simulink model "LongLatDriveline"  (R2024b)
settings: Solver=FixedStepAuto  StartTime=0  StopTime=120  FixedStep=0.002  RelTol=1e-3
InitFcn:
  | load('waypoints.mat');
  | VehicleObj = Simulink.data.dictionary.open('./ModelData/VehicleData.sldd');
  | %dDataSectObj = getSection(myDictionaryObj,'Design Data');
StopFcn:
  | Plot_LateralModelErrorControl;
  | 
  | mdlWks = get_param(gcs, 'ModelWorkspace');
  | par_ToDrvDesigner = evalin(mdlWks, 'ToDrvDesigner');
  | 
  | if par_ToDrvDesigner.Value
  |     ExportdrivingScenario;
  | end
model workspace (MAT data in the model file):
  ToDrvDesigner : Simulink.Parameter (value not decoded)
values from neighbouring files (symbols this model uses):
  A_F = 2.341157    [VehicleData.sldd]
  C_af = 80000.0    [VehicleData.sldd]
  C_ar = 80000.0    [VehicleData.sldd]
  C_d = 0.24    [VehicleData.sldd]
  f = 0.01    [VehicleData.sldd]
  g = 9.81    [VehicleData.sldd]
  h_aero = 0.65    [VehicleData.sldd]
  h_gc = 0.65    [VehicleData.sldd]
  Iz = 2873.0    [VehicleData.sldd]
  lf = 1.1    [VehicleData.sldd]
  lr = 1.58    [VehicleData.sldd]
  m = 2238.932    [VehicleData.sldd]
  Nf = 2.0    [VehicleData.sldd]
  Nr = 2.0    [VehicleData.sldd]
  r_stat = 0.342    [VehicleData.sldd]
  r_w = 0.352    [VehicleData.sldd]
  rho = 1.225    [VehicleData.sldd]
  theta = 0.0    [VehicleData.sldd]
  transGear = 0.1027    [VehicleData.sldd]
  V_wind = 0.0    [VehicleData.sldd]
symbols that are objects in the model workspace (value not decoded): ToDrvDesigner
undefined symbols (not defined in the file or in its folder): InitialPsi, InitialX, InitialY, phi
libraries: slpidlib x14, spsMosfetLib x6, simulink x4, spsVoltageMeasurementLib x3, SignalEditorBlockLib x2, spsDCVoltageSourceLib x1, spspowerguiLib x1
(part 2 of 5)

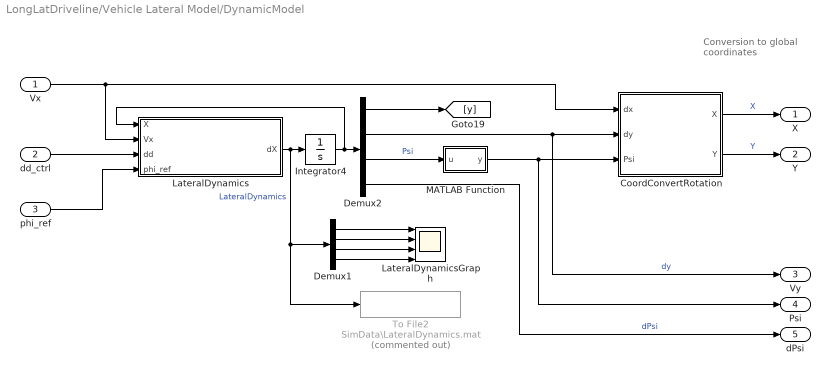
== system LongLatDriveline/Vehicle Lateral Model/DynamicModel ==
  note: Conversion to global
      | coordinates
  Vx : Inport
  dd_ctrl : Inport  Port=2
  phi_ref : Inport  Port=3
  CoordConvertRotation : Subsystem
      mask Display: image('rotatingFrame.png');
  Demux1 : Demux
  Demux2 : Demux
  Integrator4 : Integrator  InitialCondition=[0;0;InitialPsi;0.0423]
  LateralDynamics : Subsystem  Variant=on  VariantControlMode=label  LabelModeActiveChoice=Not Simplified Model
  LateralDynamicsGraph : Scope  NumInputPorts=4
  MATLAB Function : MATLAB Function  TreatAsAtomicUnit=on
  To File2 : ToFile  Commented=on  Filename=SimData\LateralDynamics.mat  SaveFormat=Timeseries
  X : Outport
  Y : Outport  Port=2
  Vy : Outport  Port=3
  Psi : Outport  Port=4
  dPsi : Outport  Port=5
  wires:
  Integrator4/1 -> LateralDynamics/1(X), Demux2/1
  phi_ref/1 -> LateralDynamics/4(phi_ref)
  Demux2/2 -> Vy/1, CoordConvertRotation/2(dy)  "dy"
  Demux1/1 -> LateralDynamicsGraph/1
  LateralDynamics/1(dX) -> To File2/1, Demux1/1, Integrator4/1  "LateralDynamics"
  Demux2/3 -> MATLAB Function/1(u)  "Psi"
  Vx/1 -> CoordConvertRotation/1(dx), LateralDynamics/2(Vx)
  Demux1/2 -> LateralDynamicsGraph/2
  CoordConvertRotation/1(X) -> X/1  "X"
  Demux1/4 -> LateralDynamicsGraph/4
  Demux2/1 -> [y]
  Demux1/3 -> LateralDynamicsGraph/3
  CoordConvertRotation/2(Y) -> Y/1  "Y"
  dd_ctrl/1 -> LateralDynamics/3(dd)
  MATLAB Function/1(y) -> CoordConvertRotation/3(Psi), Psi/1
  Demux2/4 -> dPsi/1  "dPsi"

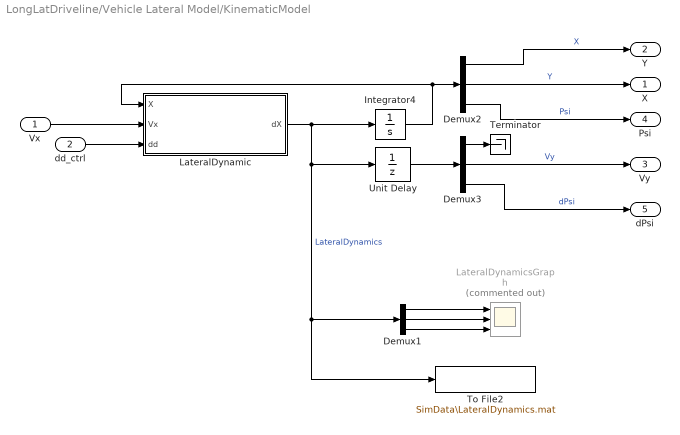
== system LongLatDriveline/Vehicle Lateral Model/KinematicModel ==
  Vx : Inport
  dd_ctrl : Inport  Port=2
  Demux1 : Demux  Outputs=3
  Demux2 : Demux  Outputs=3
  Demux3 : Demux  Outputs=3
  Integrator4 : Integrator  InitialCondition=[InitialY;InitialX;InitialPsi]
  LateralDynamic : MATLAB Function  TreatAsAtomicUnit=on  VariantControl=Simplified Model
  LateralDynamicsGraph : Scope  Commented=on  NumInputPorts=3
  Terminator : Terminator
  To File2 : ToFile  Filename=SimData\LateralDynamics.mat  SaveFormat=Timeseries
  Unit Delay : UnitDelay  InitialCondition=[0;0;0]  SampleTime=-1  HasFrameUpgradeWarning=on
  X : Outport
  Y : Outport  Port=2
  Vy : Outport  Port=3
  Psi : Outport  Port=4
  dPsi : Outport  Port=5
  wires:
  Integrator4/1 -> LateralDynamic/1(X), Demux2/1
  Vx/1 -> LateralDynamic/2(Vx)
  Demux1/1 -> LateralDynamicsGraph/1
  dd_ctrl/1 -> LateralDynamic/3(dd)
  LateralDynamic/1(dX) -> Integrator4/1, Unit Delay/1, Demux1/1, To File2/1  "LateralDynamics"
  Demux1/3 -> LateralDynamicsGraph/3
  Demux1/2 -> LateralDynamicsGraph/2
  Demux2/1 -> Y/1  "X"
  Demux2/2 -> X/1  "Y"
  Demux2/3 -> Psi/1  "Psi"
  Demux3/3 -> dPsi/1  "dPsi"
  Demux3/2 -> Vy/1  "Vy"
  Demux3/1 -> Terminator/1
  Unit Delay/1 -> Demux3/1

== system LongLatDriveline/LateralController/SMC_Alcala/LevantDiff ==
  X : Inport
  Constant : Constant  Value=lambda1
  Constant1 : Constant  Value=alpha1
  Demux : Demux  Outputs=2
  Integrator : Integrator  InitialCondition=[0 0]
  Levant : MATLAB Function  TreatAsAtomicUnit=on
  Terminator : Terminator
  dX : Outport  VectorParamsAs1DForOutWhenUnconnected=off
  wires:
  X/1 -> Levant/2(u_ref)
  Levant/1(dX) -> Integrator/1, Demux/1
  Integrator/1 -> Levant/1(X)
  Constant/1 -> Levant/3(lambda)
  Constant1/1 -> Levant/4(alpha)
  Demux/1 -> dX/1
  Demux/2 -> Terminator/1

== system LongLatDriveline/LateralController/SMC_Alcala/LevantDiff1 ==
  X : Inport
  Constant : Constant  Value=lambda1
  Constant1 : Constant  Value=alpha1
  Demux : Demux  Outputs=2
  Integrator : Integrator  InitialCondition=[0 0]
  Levant : MATLAB Function  TreatAsAtomicUnit=on
  Terminator : Terminator
  dX : Outport  VectorParamsAs1DForOutWhenUnconnected=off
  wires:
  X/1 -> Levant/2(u_ref)
  Levant/1(dX) -> Integrator/1, Demux/1
  Integrator/1 -> Levant/1(X)
  Constant/1 -> Levant/3(lambda)
  Constant1/1 -> Levant/4(alpha)
  Demux/1 -> dX/1
  Demux/2 -> Terminator/1

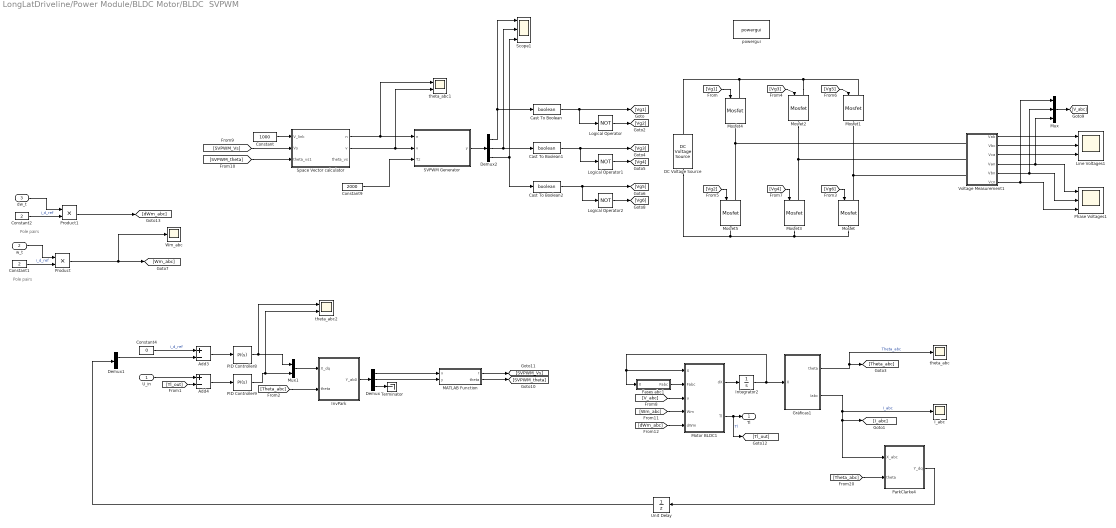
== system LongLatDriveline/Power Module/BLDC Motor/BLDC  SVPWM ==
  note: Pole pairs
  note: Pole pairs
  U_in : Inport
  w_t : Inport  Port=2
  dw_t : Inport  Port=3
  Add3 : Sum  Inputs=+-
  Add4 : Sum  Inputs=+-
  Cast To Boolean : DataTypeConversion  OutDataTypeStr=boolean  SaturateOnIntegerOverflow=off  RndMeth=Floor
  Cast To Boolean1 : DataTypeConversion  OutDataTypeStr=boolean  SaturateOnIntegerOverflow=off  RndMeth=Floor
  Cast To Boolean2 : DataTypeConversion  OutDataTypeStr=boolean  SaturateOnIntegerOverflow=off  RndMeth=Floor
  Constant : Constant  Value=1000
  Constant1 : Constant  Value=2
  Constant2 : Constant  Value=2
  Constant4 : Constant  Value=0
  Constant9 : Constant  Value=2000
  DC Voltage Source : spsDCVoltageSourceLib/DC Voltage Source  Amplitude=1000  Measurements=None
  Demux : Demux  Outputs=3
  Demux1 : Demux  Outputs=2
  Demux2 : Demux  Outputs=3
  Fases abc1 : MATLAB Function  TreatAsAtomicUnit=on
  Gráficas1 : MATLAB Function  TreatAsAtomicUnit=on
  I_abc : Scope
  Integrator2 : Integrator  InitialCondition=[0 0 0 0]
  InvPark : MATLAB Function  TreatAsAtomicUnit=on
  Line Voltages1 : Scope  NumInputPorts=3
  Logical Operator : Logic  Operator=NOT  IconShape=distinctive  AllPortsSameDT=off  OutDataTypeStr=boolean
  Logical Operator1 : Logic  Operator=NOT  IconShape=distinctive  AllPortsSameDT=off  OutDataTypeStr=boolean
  Logical Operator2 : Logic  Operator=NOT  IconShape=distinctive  AllPortsSameDT=off  OutDataTypeStr=boolean
  MATLAB Function : MATLAB Function  TreatAsAtomicUnit=on
  Mosfet{,1..5} (6 alike) : spsMosfetLib/Mosfet  Ron=0.1  Lon=0  Rd=0.01  Vfd=0  IC=0  Rs=1e5  Cs=inf  Measurements=off
  Motor BLDC1 : MATLAB Function  TreatAsAtomicUnit=on
  Mux : Mux  Inputs=3
  Mux1 : Mux  Inputs=2
  PID Controller8 : slpidlib/PID Controller  Controller=PI  Form=Parallel  TimeDomain=Continuous-time  UseExternalTs=off  SampleTime=-1  IntegratorMethod=Forward Euler  FilterMethod=Forward Euler  ControllerParametersSource=internal  P=0.203768519261034  I=30.7991199051557  UseKiTs=off  D=-6.74177637974606e-05  UseExternalDerivativeSource=off  N=1209.06435302465  UseFilter=on  TunerSelectOption=Transfer Function Based (PID Tuner App)  InitialConditionSource=internal  InitialConditionForIntegrator=0  InitialConditionForFilter=0  DifferentiatorICPrevScaledInput=0  ExternalReset=none  TrackingMode=off  Kt=1  LimitOutput=off  SatLimitsSource=internal  UpperSaturationLimit=inf  LowerSaturationLimit=-inf  LinearizeAsGain=on  AntiWindupMode=none  Kb=1  LimitIntegrator=off  UpperIntegratorSaturationLimit=inf  LowerIntegratorSaturationLimit=-inf  POutMin=[]  POutMax=[]  IOutMin=[]  IOutMax=[]  DOutMin=[]  DOutMax=[]  NOutMin=[]  NOutMax=[]  SumOutMin=[]  SumOutMax=[]  SaturationOutMin=[]  SaturationOutMax=[]  PParamMin=[]  PParamMax=[]  IParamMin=[]  IParamMax=[]  DParamMin=[]  DParamMax=[]  NParamMin=[]  NParamMax=[]  KbParamMin=[]  KbParamMax=[]  KtParamMin=[]  KtParamMax=[]  KbOutMin=[]  KbOutMax=[]  KtOutMin=[]  KtOutMax=[]  IntegratorOutMin=[]  IntegratorOutMax=[]  FilterOutMin=[]  FilterOutMax=[]  SumI1OutMin=[]  SumI1OutMax=[]  SumI2OutMin=[]  SumI2OutMax=[]  SumI3OutMin=[]  SumI3OutMax=[]  SumI4OutMin=[]  SumI4OutMax=[]  SumDOutMin=[]  SumDOutMax=[]  DifferentiatorOutMin=[]  DifferentiatorOutMax=[]  FilterDiffOutCoefMin=[]  FilterDiffOutCoefMax=[]  ReciprocalOutMin=[]  ReciprocalOutMax=[]  SumDenOutMin=[]  SumDenOutMax=[]  SumNumOutMin=[]  SumNumOutMax=[]  DivideOutMin=[]  DivideOutMax=[]  UdiffTsProdOutMin=[]  UdiffTsProdOutMax=[]  NTsProdOutMin=[]  NTsProdOutMax=[]  UintegralTsProdOutMin=[]  UintegralTsProdOutMax=[]  UngainTsProdOutMin=[]  UngainTsProdOutMax=[]  ClampingZeroOutDataTypeStr=Inherit: Inherit via back propagation  ClampingZeroOutMin=[]  ClampingZeroOutMax=[]  FilterDenConstantOutDataTypeStr=Inherit: Inherit via back propagation  FilterDenConstantOutMin=[]  FilterDenConstantOutMax=[]  PCopyOutDataTypeStr=Inherit: Inherit via back propagation  PCopyOutMin=[]  PCopyOutMax=[]  NCopyOutDataTypeStr=Inherit: Inherit via back propagation  NCopyOutMin=[]  NCopyOutMax=[]  IntegratorContinuousStateAttributes=''  IntegratorStateMustResolveToSignalObject=off  IntegratorRTWStateStorageClass=Auto  FilterContinuousStateAttributes=''  FilterStateMustResolveToSignalObject=off  FilterRTWStateStorageClass=Auto  ParallelPVariant=InternalParameters  IdealPVariant=Disabled  IVariant=InternalParameters  DVariant=Disabled  IntegratorVariant=Continuous  SatVariant=Disabled  AWVariant=Passthrough  PCopyVariant=Disabled  TRVariant=Disabled  FdbkBlocksVariant=Forward  IdealPFdbkVariant=Disabled  SatFdbkVariant=Disabled  DerivativeFilterVariant=Disabled  NVariant=Disabled  NCopyVariant=Disabled_SignalSpec  FilterICVariant=Disabled  IntegratorICVariant=InternalICs  ExternalResetVariant=Disabled  TRSumVariant=Passthrough  SumFdbkVariant=Disabled  SumVariant=Sum_PI  TsampFilterVariant=InternalTs  TsampNgainVariant=Passthrough  TsampIntegralVariant=Disabled_SignalSpec  ExternalSaturationOutDataTypeStr=Inherit: Same as second input  DerivativeSourceVariant=Disabled  PreIntVariant=InternalPreInt
  PID Controller9 : slpidlib/PID Controller  Controller=PI  Form=Parallel  TimeDomain=Continuous-time  UseExternalTs=off  SampleTime=-1  IntegratorMethod=Forward Euler  FilterMethod=Forward Euler  ControllerParametersSource=internal  P=0.203768519261034  I=30.7991199051557  UseKiTs=off  D=-6.74177637974606e-05  UseExternalDerivativeSource=off  N=1209.06435302465  UseFilter=on  TunerSelectOption=Transfer Function Based (PID Tuner App)  InitialConditionSource=internal  InitialConditionForIntegrator=0  InitialConditionForFilter=0  DifferentiatorICPrevScaledInput=0  ExternalReset=none  TrackingMode=off  Kt=1  LimitOutput=off  SatLimitsSource=internal  UpperSaturationLimit=inf  LowerSaturationLimit=-inf  LinearizeAsGain=on  AntiWindupMode=none  Kb=1  LimitIntegrator=off  UpperIntegratorSaturationLimit=inf  LowerIntegratorSaturationLimit=-inf  POutMin=[]  POutMax=[]  IOutMin=[]  IOutMax=[]  DOutMin=[]  DOutMax=[]  NOutMin=[]  NOutMax=[]  SumOutMin=[]  SumOutMax=[]  SaturationOutMin=[]  SaturationOutMax=[]  PParamMin=[]  PParamMax=[]  IParamMin=[]  IParamMax=[]  DParamMin=[]  DParamMax=[]  NParamMin=[]  NParamMax=[]  KbParamMin=[]  KbParamMax=[]  KtParamMin=[]  KtParamMax=[]  KbOutMin=[]  KbOutMax=[]  KtOutMin=[]  KtOutMax=[]  IntegratorOutMin=[]  IntegratorOutMax=[]  FilterOutMin=[]  FilterOutMax=[]  SumI1OutMin=[]  SumI1OutMax=[]  SumI2OutMin=[]  SumI2OutMax=[]  SumI3OutMin=[]  SumI3OutMax=[]  SumI4OutMin=[]  SumI4OutMax=[]  SumDOutMin=[]  SumDOutMax=[]  DifferentiatorOutMin=[]  DifferentiatorOutMax=[]  FilterDiffOutCoefMin=[]  FilterDiffOutCoefMax=[]  ReciprocalOutMin=[]  ReciprocalOutMax=[]  SumDenOutMin=[]  SumDenOutMax=[]  SumNumOutMin=[]  SumNumOutMax=[]  DivideOutMin=[]  DivideOutMax=[]  UdiffTsProdOutMin=[]  UdiffTsProdOutMax=[]  NTsProdOutMin=[]  NTsProdOutMax=[]  UintegralTsProdOutMin=[]  UintegralTsProdOutMax=[]  UngainTsProdOutMin=[]  UngainTsProdOutMax=[]  ClampingZeroOutDataTypeStr=Inherit: Inherit via back propagation  ClampingZeroOutMin=[]  ClampingZeroOutMax=[]  FilterDenConstantOutDataTypeStr=Inherit: Inherit via back propagation  FilterDenConstantOutMin=[]  FilterDenConstantOutMax=[]  PCopyOutDataTypeStr=Inherit: Inherit via back propagation  PCopyOutMin=[]  PCopyOutMax=[]  NCopyOutDataTypeStr=Inherit: Inherit via back propagation  NCopyOutMin=[]  NCopyOutMax=[]  IntegratorContinuousStateAttributes=''  IntegratorStateMustResolveToSignalObject=off  IntegratorRTWStateStorageClass=Auto  FilterContinuousStateAttributes=''  FilterStateMustResolveToSignalObject=off  FilterRTWStateStorageClass=Auto  ParallelPVariant=InternalParameters  IdealPVariant=Disabled  IVariant=InternalParameters  DVariant=Disabled  IntegratorVariant=Continuous  SatVariant=Disabled  AWVariant=Passthrough  PCopyVariant=Disabled  TRVariant=Disabled  FdbkBlocksVariant=Forward  IdealPFdbkVariant=Disabled  SatFdbkVariant=Disabled  DerivativeFilterVariant=Disabled  NVariant=Disabled  NCopyVariant=Disabled_SignalSpec  FilterICVariant=Disabled  IntegratorICVariant=InternalICs  ExternalResetVariant=Disabled  TRSumVariant=Passthrough  SumFdbkVariant=Disabled  SumVariant=Sum_PI  TsampFilterVariant=InternalTs  TsampNgainVariant=Passthrough  TsampIntegralVariant=Disabled_SignalSpec  ExternalSaturationOutDataTypeStr=Inherit: Same as second input  DerivativeSourceVariant=Disabled  PreIntVariant=InternalPreInt
  ParkClarke4 : MATLAB Function  TreatAsAtomicUnit=on
  Phase Voltages1 : Scope  NumInputPorts=3
  Product : Product
  Product1 : Product
  SVPWM Generator : Subsystem
  Scope1 : Scope  NumInputPorts=3
  Space Vector calculator : MATLAB Function  TreatAsAtomicUnit=on
  Terminator : Terminator
  Unit Delay : UnitDelay  SampleTime=-1  HasFrameUpgradeWarning=on
  Voltage Measurement1 : Subsystem
  Wm_abc : Scope
  powergui : spspowerguiLib/powergui  Priority=1  SimulationMode=Discrete  SampleTime=2e-6  frequency=60  Iterations=50  frequencyindice=0  Pbase=100e6  ErrMax=1e-4  UnitsV=kV  UnitsW=MW  buscounter=0  FunctionMessages=off  echomessages=off  EnableUseOfTLC=off  CurrentSourceSwitches=off  DisableSnubberDevices=off  DisableRonSwitches=off  DisableVfSwitches=off  DisplayEquations=off  AutomaticDiscreteSolvers=off  SolverType=Tustin/Backward Euler (TBE)  Interpol=off  ExternalGateDelay=off  methode=off  Ts=100  x0status=blocks  SPID=off  SwTol=0  HookPort=off  NonlinearTolerance=1e-4  nMaxIteration=100  ContinueOnMaxIteration=off  RestoreLinks=warning  ResistiveCurrentMeasurement=off  Frange=[0:2:500]  Ylog=off  Xlog=on  ShowGrid=off  save=off  variable=ZData  structure=ScopeData3  ZoomFFT=off  StartTime=0.04  cycles=1  DisplayStyle=1  fundamental=50  FreqAxis=off  MaxFrequency=2000  frequencyindicesteady=1  RmsSteady=1  display=off
  theta_abc : Scope
  theta_abc1 : Scope  NumInputPorts=2
  theta_abc2 : Scope  NumInputPorts=2
  Tl : Outport
  wires:
  MATLAB Function/2(theta) -> [SVPWM_theta]
  Voltage Measurement1/6(Vcn) -> Mux/1, Phase Voltages1/3
  Demux/1 -> MATLAB Function/1(x)
  Add4/1 -> PID Controller9/1
  Space Vector calculator/2(v) -> SVPWM Generator/2(v), theta_abc1/2
  Demux1/1 -> Add3/2
  [SVPWM_Vs] -> Space Vector calculator/2(Vs)
  Cast To Boolean/1 -> Logical Operator/1, [Vg1]
  SVPWM Generator/1(y) -> Demux2/1
  Logical Operator2/1 -> [Vg6]
  [SVPWM_theta] -> Space Vector calculator/3(theta_vs1)
  Cast To Boolean1/1 -> Logical Operator1/1, [Vg3]
  MATLAB Function/1(r) -> [SVPWM_Vs]
  Voltage Measurement1/2(Vbc) -> Line Voltages1/2
  Mux1/1 -> InvPark/1(X_dq)
  Logical Operator/1 -> [Vg2]
  Logical Operator1/1 -> [Vg4]
  [Theta_abc] -> InvPark/2(theta)
  Demux/3 -> Terminator/1
  Cast To Boolean2/1 -> Logical Operator2/1, [Vg5]
  Demux2/1 -> Cast To Boolean/1, Scope1/1
  [Vg2] -> Mosfet5/1
  Demux/2 -> MATLAB Function/2(y)
  [Vg1] -> Mosfet4/1
  Constant/1 -> Space Vector calculator/1(V_link)
  Mux/1 -> [V_abc]
  Gráficas1/2(Iabc) -> ParkClarke4/1(X_abc), [I_abc], I_abc/1  "I_abc"
  Voltage Measurement1/4(Van) -> Mux/3, Phase Voltages1/1
  Voltage Measurement1/5(Vbn) -> Mux/2, Phase Voltages1/2
  [Vg3] -> Mosfet2/1
  [Vg5] -> Mosfet1/1
  Space Vector calculator/1(n) -> SVPWM Generator/1(n), theta_abc1/1
  Constant9/1 -> SVPWM Generator/3(Tz)
  ParkClarke4/1(Y_dq) -> Unit Delay/1
  Demux2/3 -> Cast To Boolean2/1, Scope1/3
  [Vg6] -> Mosfet/1
  Voltage Measurement1/3(Vca) -> Line Voltages1/3
  Demux2/2 -> Cast To Boolean1/1, Scope1/2
  [Theta_abc] -> ParkClarke4/2(theta)
  Gráficas1/1(theta) -> theta_abc/1, [Theta_abc]  "Theta_abc"
  [Vg4] -> Mosfet3/1
  Voltage Measurement1/1(Vab) -> Line Voltages1/1
  Add3/1 -> PID Controller8/1
  Unit Delay/1 -> Demux1/1
  PID Controller9/1 -> Mux1/2, theta_abc2/2
  PID Controller8/1 -> Mux1/1, theta_abc2/1
  Integrator2/1 -> Gráficas1/1(X), Motor BLDC1/1(X), Fases abc1/1(X)
  Constant4/1 -> Add3/1  "i_d_ref"
  InvPark/1(Y_ab0) -> Demux/1
  Motor BLDC1/1(dX) -> Integrator2/1
  [V_abc] -> Motor BLDC1/3(u)
  Fases abc1/1(Fabc) -> Motor BLDC1/2(Fabc)
  Motor BLDC1/2(Tl) -> [Tl_out], Tl/1  "Tl"
  [Wm_abc] -> Motor BLDC1/4(Wm)
  U_in/1 -> Add4/1
  [Tl_out] -> Add4/2
  w_t/1 -> Product/1
  Constant1/1 -> Product/2  "i_d_ref"
  Product/1 -> Wm_abc/1, [Wm_abc]
  Constant2/1 -> Product1/2  "i_d_ref"
  dw_t/1 -> Product1/1
  Product1/1 -> [dWm_abc]
  [dWm_abc] -> Motor BLDC1/5(dWm)
  connections:
  DC Voltage Source/LConn1 -- Mosfet3/RConn1 -- Mosfet/RConn1 -- Mosfet5/RConn1
  Mosfet4/RConn1 -- Mosfet5/LConn1 -- Voltage Measurement1/LConn1
  Mosfet2/LConn1 -- Mosfet1/LConn1 -- DC Voltage Source/RConn1 -- Mosfet4/LConn1
  Mosfet1/RConn1 -- Voltage Measurement1/LConn3 -- Mosfet/LConn1
  Mosfet2/RConn1 -- Voltage Measurement1/LConn2 -- Mosfet3/LConn1

== system LongLatDriveline/Power Module/BLDC Motor/BLDC abcModel ==
  U_in : Inport
  w_t : Inport  Port=2
  dw_t : Inport  Port=3
  Fases abc : MATLAB Function  TreatAsAtomicUnit=on
  Graphs : MATLAB Function  TreatAsAtomicUnit=on
  Iabc : Scope
  Integrator2 : Integrator  InitialCondition=[0 0 0 0]
  Motor BLDC : MATLAB Function  TreatAsAtomicUnit=on
  theta : Scope
  Tl : Outport
  wires:
  Graphs/1(theta) -> theta/1
  Graphs/2(Iabc) -> Iabc/1
  Fases abc/1(Fabc) -> Motor BLDC/2(Fabc)
  Motor BLDC/1(dX) -> Integrator2/1
  Integrator2/1 -> Graphs/1(X), Motor BLDC/1(X), Fases abc/1(X)
  Motor BLDC/2(Tl) -> Tl/1  "Tl"
  dw_t/1 -> Motor BLDC/5(dWm)
  w_t/1 -> Motor BLDC/4(Wm)
  U_in/1 -> Motor BLDC/3(u)  "i_q_ref"

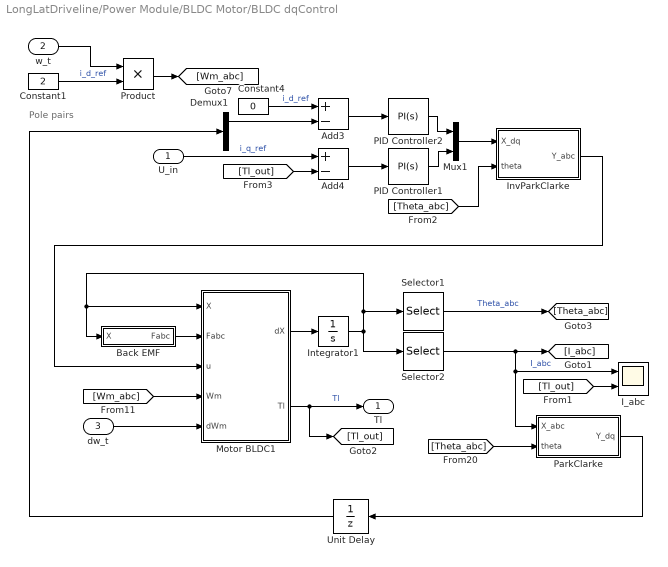
== system LongLatDriveline/Power Module/BLDC Motor/BLDC dqControl ==
  note: Pole pairs
  U_in : Inport
  w_t : Inport  Port=2
  dw_t : Inport  Port=3
  Add3 : Sum  Inputs=+-
  Add4 : Sum  Inputs=+-
  Back EMF : MATLAB Function  TreatAsAtomicUnit=on
  Constant1 : Constant  Value=2
  Constant4 : Constant  Value=0
  Demux1 : Demux  Outputs=2
  I_abc : Scope  NumInputPorts=2
  Integrator1 : Integrator  InitialCondition=[0;0;0;0]
  InvParkClarke : MATLAB Function  TreatAsAtomicUnit=on
  Motor BLDC1 : MATLAB Function  TreatAsAtomicUnit=on
  Mux1 : Mux  Inputs=2
  PID Controller1 : slpidlib/PID Controller  Controller=PI  Form=Parallel  TimeDomain=Continuous-time  UseExternalTs=off  SampleTime=-1  IntegratorMethod=Forward Euler  FilterMethod=Forward Euler  ControllerParametersSource=internal  P=-1.56443937452264  I=-236.594680688707  UseKiTs=off  D=0  UseExternalDerivativeSource=off  N=100  UseFilter=on  TunerSelectOption=Transfer Function Based (PID Tuner App)  InitialConditionSource=internal  InitialConditionForIntegrator=0  InitialConditionForFilter=0  DifferentiatorICPrevScaledInput=0  ExternalReset=none  TrackingMode=off  Kt=1  LimitOutput=off  SatLimitsSource=internal  UpperSaturationLimit=inf  LowerSaturationLimit=-inf  LinearizeAsGain=on  AntiWindupMode=none  Kb=1  LimitIntegrator=off  UpperIntegratorSaturationLimit=inf  LowerIntegratorSaturationLimit=-inf  POutMin=[]  POutMax=[]  IOutMin=[]  IOutMax=[]  DOutMin=[]  DOutMax=[]  NOutMin=[]  NOutMax=[]  SumOutMin=[]  SumOutMax=[]  SaturationOutMin=[]  SaturationOutMax=[]  PParamMin=[]  PParamMax=[]  IParamMin=[]  IParamMax=[]  DParamMin=[]  DParamMax=[]  NParamMin=[]  NParamMax=[]  KbParamMin=[]  KbParamMax=[]  KtParamMin=[]  KtParamMax=[]  KbOutMin=[]  KbOutMax=[]  KtOutMin=[]  KtOutMax=[]  IntegratorOutMin=[]  IntegratorOutMax=[]  FilterOutMin=[]  FilterOutMax=[]  SumI1OutMin=[]  SumI1OutMax=[]  SumI2OutMin=[]  SumI2OutMax=[]  SumI3OutMin=[]  SumI3OutMax=[]  SumI4OutMin=[]  SumI4OutMax=[]  SumDOutMin=[]  SumDOutMax=[]  DifferentiatorOutMin=[]  DifferentiatorOutMax=[]  FilterDiffOutCoefMin=[]  FilterDiffOutCoefMax=[]  ReciprocalOutMin=[]  ReciprocalOutMax=[]  SumDenOutMin=[]  SumDenOutMax=[]  SumNumOutMin=[]  SumNumOutMax=[]  DivideOutMin=[]  DivideOutMax=[]  UdiffTsProdOutMin=[]  UdiffTsProdOutMax=[]  NTsProdOutMin=[]  NTsProdOutMax=[]  UintegralTsProdOutMin=[]  UintegralTsProdOutMax=[]  UngainTsProdOutMin=[]  UngainTsProdOutMax=[]  ClampingZeroOutDataTypeStr=Inherit: Inherit via back propagation  ClampingZeroOutMin=[]  ClampingZeroOutMax=[]  FilterDenConstantOutDataTypeStr=Inherit: Inherit via back propagation  FilterDenConstantOutMin=[]  FilterDenConstantOutMax=[]  PCopyOutDataTypeStr=Inherit: Inherit via back propagation  PCopyOutMin=[]  PCopyOutMax=[]  NCopyOutDataTypeStr=Inherit: Inherit via back propagation  NCopyOutMin=[]  NCopyOutMax=[]  IntegratorContinuousStateAttributes=''  IntegratorStateMustResolveToSignalObject=off  IntegratorRTWStateStorageClass=Auto  FilterContinuousStateAttributes=''  FilterStateMustResolveToSignalObject=off  FilterRTWStateStorageClass=Auto  ParallelPVariant=InternalParameters  IdealPVariant=Disabled  IVariant=InternalParameters  DVariant=Disabled  IntegratorVariant=Continuous  SatVariant=Disabled  AWVariant=Passthrough  PCopyVariant=Disabled  TRVariant=Disabled  FdbkBlocksVariant=Forward  IdealPFdbkVariant=Disabled  SatFdbkVariant=Disabled  DerivativeFilterVariant=Disabled  NVariant=Disabled  NCopyVariant=Disabled_SignalSpec  FilterICVariant=Disabled  IntegratorICVariant=InternalICs  ExternalResetVariant=Disabled  TRSumVariant=Passthrough  SumFdbkVariant=Disabled  SumVariant=Sum_PI  TsampFilterVariant=InternalTs  TsampNgainVariant=Passthrough  TsampIntegralVariant=Disabled_SignalSpec  ExternalSaturationOutDataTypeStr=Inherit: Same as second input  DerivativeSourceVariant=Disabled  PreIntVariant=InternalPreInt
  PID Controller2 : slpidlib/PID Controller  Controller=PI  Form=Parallel  TimeDomain=Continuous-time  UseExternalTs=off  SampleTime=-1  IntegratorMethod=Forward Euler  FilterMethod=Forward Euler  ControllerParametersSource=internal  P=0.214157493658236  I=32.3133576614742  UseKiTs=off  D=0  UseExternalDerivativeSource=off  N=100  UseFilter=on  TunerSelectOption=Transfer Function Based (PID Tuner App)  InitialConditionSource=internal  InitialConditionForIntegrator=0  InitialConditionForFilter=0  DifferentiatorICPrevScaledInput=0  ExternalReset=none  TrackingMode=off  Kt=1  LimitOutput=off  SatLimitsSource=internal  UpperSaturationLimit=inf  LowerSaturationLimit=-inf  LinearizeAsGain=on  AntiWindupMode=none  Kb=1  LimitIntegrator=off  UpperIntegratorSaturationLimit=inf  LowerIntegratorSaturationLimit=-inf  POutMin=[]  POutMax=[]  IOutMin=[]  IOutMax=[]  DOutMin=[]  DOutMax=[]  NOutMin=[]  NOutMax=[]  SumOutMin=[]  SumOutMax=[]  SaturationOutMin=[]  SaturationOutMax=[]  PParamMin=[]  PParamMax=[]  IParamMin=[]  IParamMax=[]  DParamMin=[]  DParamMax=[]  NParamMin=[]  NParamMax=[]  KbParamMin=[]  KbParamMax=[]  KtParamMin=[]  KtParamMax=[]  KbOutMin=[]  KbOutMax=[]  KtOutMin=[]  KtOutMax=[]  IntegratorOutMin=[]  IntegratorOutMax=[]  FilterOutMin=[]  FilterOutMax=[]  SumI1OutMin=[]  SumI1OutMax=[]  SumI2OutMin=[]  SumI2OutMax=[]  SumI3OutMin=[]  SumI3OutMax=[]  SumI4OutMin=[]  SumI4OutMax=[]  SumDOutMin=[]  SumDOutMax=[]  DifferentiatorOutMin=[]  DifferentiatorOutMax=[]  FilterDiffOutCoefMin=[]  FilterDiffOutCoefMax=[]  ReciprocalOutMin=[]  ReciprocalOutMax=[]  SumDenOutMin=[]  SumDenOutMax=[]  SumNumOutMin=[]  SumNumOutMax=[]  DivideOutMin=[]  DivideOutMax=[]  UdiffTsProdOutMin=[]  UdiffTsProdOutMax=[]  NTsProdOutMin=[]  NTsProdOutMax=[]  UintegralTsProdOutMin=[]  UintegralTsProdOutMax=[]  UngainTsProdOutMin=[]  UngainTsProdOutMax=[]  ClampingZeroOutDataTypeStr=Inherit: Inherit via back propagation  ClampingZeroOutMin=[]  ClampingZeroOutMax=[]  FilterDenConstantOutDataTypeStr=Inherit: Inherit via back propagation  FilterDenConstantOutMin=[]  FilterDenConstantOutMax=[]  PCopyOutDataTypeStr=Inherit: Inherit via back propagation  PCopyOutMin=[]  PCopyOutMax=[]  NCopyOutDataTypeStr=Inherit: Inherit via back propagation  NCopyOutMin=[]  NCopyOutMax=[]  IntegratorContinuousStateAttributes=''  IntegratorStateMustResolveToSignalObject=off  IntegratorRTWStateStorageClass=Auto  FilterContinuousStateAttributes=''  FilterStateMustResolveToSignalObject=off  FilterRTWStateStorageClass=Auto  ParallelPVariant=InternalParameters  IdealPVariant=Disabled  IVariant=InternalParameters  DVariant=Disabled  IntegratorVariant=Continuous  SatVariant=Disabled  AWVariant=Passthrough  PCopyVariant=Disabled  TRVariant=Disabled  FdbkBlocksVariant=Forward  IdealPFdbkVariant=Disabled  SatFdbkVariant=Disabled  DerivativeFilterVariant=Disabled  NVariant=Disabled  NCopyVariant=Disabled_SignalSpec  FilterICVariant=Disabled  IntegratorICVariant=InternalICs  ExternalResetVariant=Disabled  TRSumVariant=Passthrough  SumFdbkVariant=Disabled  SumVariant=Sum_PI  TsampFilterVariant=InternalTs  TsampNgainVariant=Passthrough  TsampIntegralVariant=Disabled_SignalSpec  ExternalSaturationOutDataTypeStr=Inherit: Same as second input  DerivativeSourceVariant=Disabled  PreIntVariant=InternalPreInt
  ParkClarke : MATLAB Function  TreatAsAtomicUnit=on
  Product : Product
  Selector1 : Selector  InputPortWidth=4  IndexOptions=Index vector (dialog)  Indices=[1]  OutputSizes=1
  Selector2 : Selector  InputPortWidth=4  IndexOptions=Index vector (dialog)  Indices=[2:4]  OutputSizes=1
  Unit Delay : UnitDelay  InitialCondition=[0;0]  SampleTime=-1  HasFrameUpgradeWarning=on
  Tl : Outport
  wires:
  Constant4/1 -> Add3/1  "i_d_ref"
  [Theta_abc] -> ParkClarke/2(theta)
  Motor BLDC1/2(Tl) -> [Tl_out], Tl/1  "Tl"
  Selector2/1 -> [I_abc], ParkClarke/1(X_abc), I_abc/1  "I_abc"
  Add4/1 -> PID Controller1/1
  InvParkClarke/1(Y_abc) -> Motor BLDC1/3(u)
  Motor BLDC1/1(dX) -> Integrator1/1
  Demux1/1 -> Add3/2
  [Wm_abc] -> Motor BLDC1/4(Wm)
  Back EMF/1(Fabc) -> Motor BLDC1/2(Fabc)
  Add3/1 -> PID Controller2/1
  ParkClarke/1(Y_dq) -> Unit Delay/1
  PID Controller1/1 -> Mux1/2
  U_in/1 -> Add4/1  "i_q_ref"
  dw_t/1 -> Motor BLDC1/5(dWm)
  PID Controller2/1 -> Mux1/1
  Selector1/1 -> [Theta_abc]  "Theta_abc"
  [Tl_out] -> Add4/2
  Integrator1/1 -> Selector1/1, Back EMF/1(X), Motor BLDC1/1(X), Selector2/1
  [Theta_abc] -> InvParkClarke/2(theta)
  Mux1/1 -> InvParkClarke/1(X_dq)
  Unit Delay/1 -> Demux1/1
  Constant1/1 -> Product/2  "i_d_ref"
  Product/1 -> [Wm_abc]
  w_t/1 -> Product/1
  [Tl_out] -> I_abc/2

== system LongLatDriveline/Power Module/SIEngineModel/SI_Engine ==
  p_man : Inport
  T_man : Inport  Port=2
  alpha : Inport  Port=3
  w_e : Inport  Port=4
  dw_e : Inport  Port=5
  Add : Sum  Inputs=+--
  Add1 : Sum  Inputs=-+
  Constant15 : Constant  Value=.6
  Divide : Product  Inputs=**
  FrictionLosses : MATLAB Function  TreatAsAtomicUnit=on
  InflowRateManifold : MATLAB Function  TreatAsAtomicUnit=on
  Integrator1 : Integrator
  ManifoldPressure : MATLAB Function  TreatAsAtomicUnit=on
  OutflowRateManifold : MATLAB Function  TreatAsAtomicUnit=on
  indTorque : MATLAB Function  TreatAsAtomicUnit=on
  T_p : Outport  VectorParamsAs1DForOutWhenUnconnected=off
  wires:
  ManifoldPressure/1(dp_man) -> FrictionLosses/2(p_man)
  InflowRateManifold/1(dm_ai) -> Add1/2, ManifoldPressure/2(dm_ai)
  OutflowRateManifold/1(dm_ao) -> Add1/1, ManifoldPressure/1(dm_ao), indTorque/2(dm_ao)
  indTorque/1(T_ind) -> Add/1
  p_man/1 -> InflowRateManifold/2(p_man), OutflowRateManifold/2(p_man)
  FrictionLosses/1(T_f) -> Add/2
  alpha/1 -> InflowRateManifold/1(alpha)
  Add1/1 -> Integrator1/1
  Integrator1/1 -> OutflowRateManifold/4(ma)
  T_man/1 -> OutflowRateManifold/3(T_man)
  w_e/1 -> FrictionLosses/1(w_e), indTorque/1(w_e), OutflowRateManifold/1(w_e)
  Constant15/1 -> Divide/1
  dw_e/1 -> Divide/2
  Divide/1 -> Add/3
  Add/1 -> T_p/1

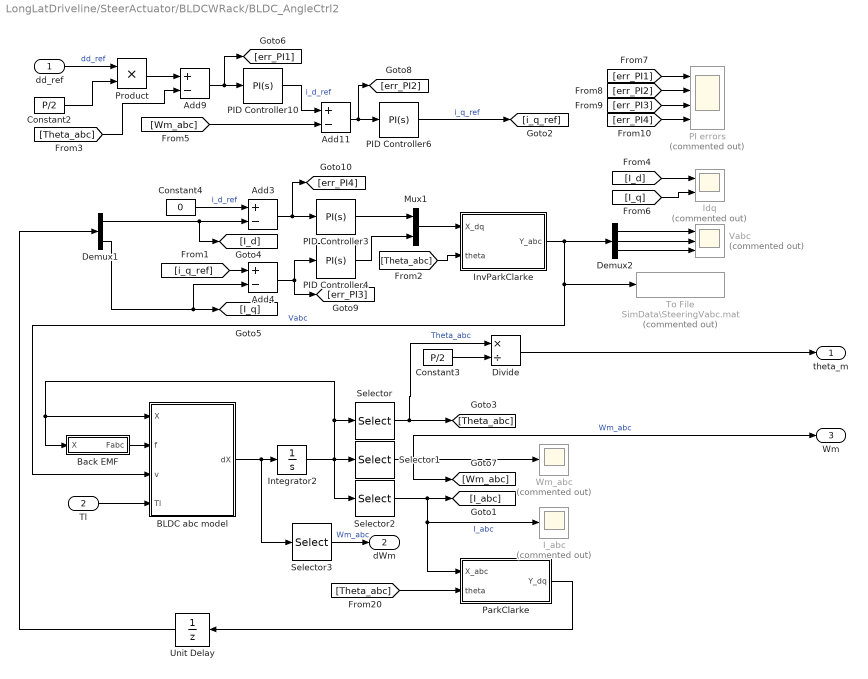
== system LongLatDriveline/SteerActuator/BLDCWRack/BLDC_AngleCtrl2 ==
  dd_ref : Inport
  Tl : Inport  Port=2
  Add{3..4,9,11} (4 alike) : Sum  Inputs=+-
  BLDC abc model : MATLAB Function  TreatAsAtomicUnit=on
  Back EMF : MATLAB Function  TreatAsAtomicUnit=on
  Constant2 : Constant  Value=P/2
  Constant3 : Constant  Value=P/2
  Constant4 : Constant  Value=0
  Demux1 : Demux  Outputs=2
  Demux2 : Demux  Outputs=3
  Divide : Product  Inputs=*/
  I_abc : Scope  Commented=on
  Idq : Scope  Commented=on  NumInputPorts=2
  Integrator2 : Integrator  InitialCondition=[0;0;0;0.1;0]
  InvParkClarke : MATLAB Function  TreatAsAtomicUnit=on
  Mux1 : Mux  Inputs=2
  PI errors : Scope  Commented=on  NumInputPorts=4
  PID Controller10 : slpidlib/PID Controller  Controller=PI  Form=Parallel  TimeDomain=Continuous-time  UseExternalTs=off  SampleTime=-1  IntegratorMethod=Forward Euler  FilterMethod=Forward Euler  ControllerParametersSource=internal  P=50  I=2  UseKiTs=off  D=0  UseExternalDerivativeSource=off  N=100  UseFilter=on  TunerSelectOption=Transfer Function Based (PID Tuner App)  InitialConditionSource=internal  InitialConditionForIntegrator=0  InitialConditionForFilter=0  DifferentiatorICPrevScaledInput=0  ExternalReset=none  TrackingMode=off  Kt=1  LimitOutput=off  SatLimitsSource=internal  UpperSaturationLimit=500  LowerSaturationLimit=-500  LinearizeAsGain=on  AntiWindupMode=back-calculation  Kb=1  LimitIntegrator=off  UpperIntegratorSaturationLimit=inf  LowerIntegratorSaturationLimit=-inf  POutMin=[]  POutMax=[]  IOutMin=[]  IOutMax=[]  DOutMin=[]  DOutMax=[]  NOutMin=[]  NOutMax=[]  SumOutMin=[]  SumOutMax=[]  SaturationOutMin=[]  SaturationOutMax=[]  PParamMin=[]  PParamMax=[]  IParamMin=[]  IParamMax=[]  DParamMin=[]  DParamMax=[]  NParamMin=[]  NParamMax=[]  KbParamMin=[]  KbParamMax=[]  KtParamMin=[]  KtParamMax=[]  KbOutMin=[]  KbOutMax=[]  KtOutMin=[]  KtOutMax=[]  IntegratorOutMin=[]  IntegratorOutMax=[]  FilterOutMin=[]  FilterOutMax=[]  SumI1OutMin=[]  SumI1OutMax=[]  SumI2OutMin=[]  SumI2OutMax=[]  SumI3OutMin=[]  SumI3OutMax=[]  SumI4OutMin=[]  SumI4OutMax=[]  SumDOutMin=[]  SumDOutMax=[]  DifferentiatorOutMin=[]  DifferentiatorOutMax=[]  FilterDiffOutCoefMin=[]  FilterDiffOutCoefMax=[]  ReciprocalOutMin=[]  ReciprocalOutMax=[]  SumDenOutMin=[]  SumDenOutMax=[]  SumNumOutMin=[]  SumNumOutMax=[]  DivideOutMin=[]  DivideOutMax=[]  UdiffTsProdOutMin=[]  UdiffTsProdOutMax=[]  NTsProdOutMin=[]  NTsProdOutMax=[]  UintegralTsProdOutMin=[]  UintegralTsProdOutMax=[]  UngainTsProdOutMin=[]  UngainTsProdOutMax=[]  ClampingZeroOutDataTypeStr=Inherit: Inherit via back propagation  ClampingZeroOutMin=[]  ClampingZeroOutMax=[]  FilterDenConstantOutDataTypeStr=Inherit: Inherit via back propagation  FilterDenConstantOutMin=[]  FilterDenConstantOutMax=[]  PCopyOutDataTypeStr=Inherit: Inherit via back propagation  PCopyOutMin=[]  PCopyOutMax=[]  NCopyOutDataTypeStr=Inherit: Inherit via back propagation  NCopyOutMin=[]  NCopyOutMax=[]  IntegratorContinuousStateAttributes=''  IntegratorStateMustResolveToSignalObject=off  IntegratorRTWStateStorageClass=Auto  FilterContinuousStateAttributes=''  FilterStateMustResolveToSignalObject=off  FilterRTWStateStorageClass=Auto  ParallelPVariant=InternalParameters  IdealPVariant=Disabled  IVariant=InternalParameters  DVariant=Disabled  IntegratorVariant=Continuous  SatVariant=Disabled  AWVariant=Passthrough  PCopyVariant=Disabled  TRVariant=Disabled  FdbkBlocksVariant=Forward  IdealPFdbkVariant=Disabled  SatFdbkVariant=Disabled  DerivativeFilterVariant=Disabled  NVariant=Disabled  NCopyVariant=Disabled_SignalSpec  FilterICVariant=Disabled  IntegratorICVariant=InternalICs  ExternalResetVariant=Disabled  TRSumVariant=Passthrough  SumFdbkVariant=Disabled  SumVariant=Sum_PI  TsampFilterVariant=InternalTs  TsampNgainVariant=Passthrough  TsampIntegralVariant=Disabled_SignalSpec  ExternalSaturationOutDataTypeStr=Inherit: Same as second input  DerivativeSourceVariant=Disabled  PreIntVariant=InternalPreInt
  PID Controller3 : slpidlib/PID Controller  Controller=PI  Form=Parallel  TimeDomain=Continuous-time  UseExternalTs=off  SampleTime=-1  IntegratorMethod=Forward Euler  FilterMethod=Forward Euler  ControllerParametersSource=internal  P=30  I=0  UseKiTs=off  D=0  UseExternalDerivativeSource=off  N=100  UseFilter=on  TunerSelectOption=Transfer Function Based (PID Tuner App)  InitialConditionSource=internal  InitialConditionForIntegrator=0  InitialConditionForFilter=0  DifferentiatorICPrevScaledInput=0  ExternalReset=none  TrackingMode=off  Kt=1  LimitOutput=on  SatLimitsSource=internal  UpperSaturationLimit=sqrt(2/3)*13.5  LowerSaturationLimit=-sqrt(2/3)*13.5  LinearizeAsGain=on  AntiWindupMode=back-calculation  Kb=1  LimitIntegrator=off  UpperIntegratorSaturationLimit=inf  LowerIntegratorSaturationLimit=-inf  POutMin=[]  POutMax=[]  IOutMin=[]  IOutMax=[]  DOutMin=[]  DOutMax=[]  NOutMin=[]  NOutMax=[]  SumOutMin=[]  SumOutMax=[]  SaturationOutMin=[]  SaturationOutMax=[]  PParamMin=[]  PParamMax=[]  IParamMin=[]  IParamMax=[]  DParamMin=[]  DParamMax=[]  NParamMin=[]  NParamMax=[]  KbParamMin=[]  KbParamMax=[]  KtParamMin=[]  KtParamMax=[]  KbOutMin=[]  KbOutMax=[]  KtOutMin=[]  KtOutMax=[]  IntegratorOutMin=[]  IntegratorOutMax=[]  FilterOutMin=[]  FilterOutMax=[]  SumI1OutMin=[]  SumI1OutMax=[]  SumI2OutMin=[]  SumI2OutMax=[]  SumI3OutMin=[]  SumI3OutMax=[]  SumI4OutMin=[]  SumI4OutMax=[]  SumDOutMin=[]  SumDOutMax=[]  DifferentiatorOutMin=[]  DifferentiatorOutMax=[]  FilterDiffOutCoefMin=[]  FilterDiffOutCoefMax=[]  ReciprocalOutMin=[]  ReciprocalOutMax=[]  SumDenOutMin=[]  SumDenOutMax=[]  SumNumOutMin=[]  SumNumOutMax=[]  DivideOutMin=[]  DivideOutMax=[]  UdiffTsProdOutMin=[]  UdiffTsProdOutMax=[]  NTsProdOutMin=[]  NTsProdOutMax=[]  UintegralTsProdOutMin=[]  UintegralTsProdOutMax=[]  UngainTsProdOutMin=[]  UngainTsProdOutMax=[]  ClampingZeroOutDataTypeStr=Inherit: Inherit via back propagation  ClampingZeroOutMin=[]  ClampingZeroOutMax=[]  FilterDenConstantOutDataTypeStr=Inherit: Inherit via back propagation  FilterDenConstantOutMin=[]  FilterDenConstantOutMax=[]  PCopyOutDataTypeStr=Inherit: Inherit via back propagation  PCopyOutMin=[]  PCopyOutMax=[]  NCopyOutDataTypeStr=Inherit: Inherit via back propagation  NCopyOutMin=[]  NCopyOutMax=[]  IntegratorContinuousStateAttributes=''  IntegratorStateMustResolveToSignalObject=off  IntegratorRTWStateStorageClass=Auto  FilterContinuousStateAttributes=''  FilterStateMustResolveToSignalObject=off  FilterRTWStateStorageClass=Auto  ParallelPVariant=InternalParameters  IdealPVariant=Disabled  IVariant=InternalParameters  DVariant=Disabled  IntegratorVariant=Continuous  SatVariant=Enabled  AWVariant=BackCalculation  PCopyVariant=Disabled  TRVariant=Disabled  FdbkBlocksVariant=Forward  IdealPFdbkVariant=Disabled  SatFdbkVariant=Disabled  DerivativeFilterVariant=Disabled  NVariant=Disabled  NCopyVariant=Disabled_SignalSpec  FilterICVariant=Disabled  IntegratorICVariant=InternalICs  ExternalResetVariant=Disabled  TRSumVariant=Passthrough  SumFdbkVariant=Disabled  SumVariant=Sum_PI  TsampFilterVariant=InternalTs  TsampNgainVariant=Passthrough  TsampIntegralVariant=Disabled_SignalSpec  ExternalSaturationOutDataTypeStr=Inherit: Same as second input  DerivativeSourceVariant=Disabled  PreIntVariant=InternalPreInt
  PID Controller4 : slpidlib/PID Controller  Controller=PI  Form=Parallel  TimeDomain=Continuous-time  UseExternalTs=off  SampleTime=-1  IntegratorMethod=Forward Euler  FilterMethod=Forward Euler  ControllerParametersSource=internal  P=40  I=80  UseKiTs=off  D=0  UseExternalDerivativeSource=off  N=100  UseFilter=on  TunerSelectOption=Transfer Function Based (PID Tuner App)  InitialConditionSource=internal  InitialConditionForIntegrator=0  InitialConditionForFilter=0  DifferentiatorICPrevScaledInput=0  ExternalReset=none  TrackingMode=off  Kt=1  LimitOutput=on  SatLimitsSource=internal  UpperSaturationLimit=sqrt(2/3)*13.5  LowerSaturationLimit=-sqrt(2/3)*13.5  LinearizeAsGain=on  AntiWindupMode=back-calculation  Kb=1  LimitIntegrator=off  UpperIntegratorSaturationLimit=inf  LowerIntegratorSaturationLimit=-inf  POutMin=[]  POutMax=[]  IOutMin=[]  IOutMax=[]  DOutMin=[]  DOutMax=[]  NOutMin=[]  NOutMax=[]  SumOutMin=[]  SumOutMax=[]  SaturationOutMin=[]  SaturationOutMax=[]  PParamMin=[]  PParamMax=[]  IParamMin=[]  IParamMax=[]  DParamMin=[]  DParamMax=[]  NParamMin=[]  NParamMax=[]  KbParamMin=[]  KbParamMax=[]  KtParamMin=[]  KtParamMax=[]  KbOutMin=[]  KbOutMax=[]  KtOutMin=[]  KtOutMax=[]  IntegratorOutMin=[]  IntegratorOutMax=[]  FilterOutMin=[]  FilterOutMax=[]  SumI1OutMin=[]  SumI1OutMax=[]  SumI2OutMin=[]  SumI2OutMax=[]  SumI3OutMin=[]  SumI3OutMax=[]  SumI4OutMin=[]  SumI4OutMax=[]  SumDOutMin=[]  SumDOutMax=[]  DifferentiatorOutMin=[]  DifferentiatorOutMax=[]  FilterDiffOutCoefMin=[]  FilterDiffOutCoefMax=[]  ReciprocalOutMin=[]  ReciprocalOutMax=[]  SumDenOutMin=[]  SumDenOutMax=[]  SumNumOutMin=[]  SumNumOutMax=[]  DivideOutMin=[]  DivideOutMax=[]  UdiffTsProdOutMin=[]  UdiffTsProdOutMax=[]  NTsProdOutMin=[]  NTsProdOutMax=[]  UintegralTsProdOutMin=[]  UintegralTsProdOutMax=[]  UngainTsProdOutMin=[]  UngainTsProdOutMax=[]  ClampingZeroOutDataTypeStr=Inherit: Inherit via back propagation  ClampingZeroOutMin=[]  ClampingZeroOutMax=[]  FilterDenConstantOutDataTypeStr=Inherit: Inherit via back propagation  FilterDenConstantOutMin=[]  FilterDenConstantOutMax=[]  PCopyOutDataTypeStr=Inherit: Inherit via back propagation  PCopyOutMin=[]  PCopyOutMax=[]  NCopyOutDataTypeStr=Inherit: Inherit via back propagation  NCopyOutMin=[]  NCopyOutMax=[]  IntegratorContinuousStateAttributes=''  IntegratorStateMustResolveToSignalObject=off  IntegratorRTWStateStorageClass=Auto  FilterContinuousStateAttributes=''  FilterStateMustResolveToSignalObject=off  FilterRTWStateStorageClass=Auto  ParallelPVariant=InternalParameters  IdealPVariant=Disabled  IVariant=InternalParameters  DVariant=Disabled  IntegratorVariant=Continuous  SatVariant=Enabled  AWVariant=BackCalculation  PCopyVariant=Disabled  TRVariant=Disabled  FdbkBlocksVariant=Forward  IdealPFdbkVariant=Disabled  SatFdbkVariant=Disabled  DerivativeFilterVariant=Disabled  NVariant=Disabled  NCopyVariant=Disabled_SignalSpec  FilterICVariant=Disabled  IntegratorICVariant=InternalICs  ExternalResetVariant=Disabled  TRSumVariant=Passthrough  SumFdbkVariant=Disabled  SumVariant=Sum_PI  TsampFilterVariant=InternalTs  TsampNgainVariant=Passthrough  TsampIntegralVariant=Disabled_SignalSpec  ExternalSaturationOutDataTypeStr=Inherit: Same as second input  DerivativeSourceVariant=Disabled  PreIntVariant=InternalPreInt
  PID Controller6 : slpidlib/PID Controller  Controller=PI  Form=Parallel  TimeDomain=Continuous-time  UseExternalTs=off  SampleTime=-1  IntegratorMethod=Forward Euler  FilterMethod=Forward Euler  ControllerParametersSource=internal  P=-15  I=-75  UseKiTs=off  D=0  UseExternalDerivativeSource=off  N=100  UseFilter=on  TunerSelectOption=Transfer Function Based (PID Tuner App)  InitialConditionSource=internal  InitialConditionForIntegrator=0  InitialConditionForFilter=0  DifferentiatorICPrevScaledInput=0  ExternalReset=none  TrackingMode=off  Kt=1  LimitOutput=off  SatLimitsSource=internal  UpperSaturationLimit=500  LowerSaturationLimit=-500  LinearizeAsGain=on  AntiWindupMode=back-calculation  Kb=1  LimitIntegrator=off  UpperIntegratorSaturationLimit=inf  LowerIntegratorSaturationLimit=-inf  POutMin=[]  POutMax=[]  IOutMin=[]  IOutMax=[]  DOutMin=[]  DOutMax=[]  NOutMin=[]  NOutMax=[]  SumOutMin=[]  SumOutMax=[]  SaturationOutMin=[]  SaturationOutMax=[]  PParamMin=[]  PParamMax=[]  IParamMin=[]  IParamMax=[]  DParamMin=[]  DParamMax=[]  NParamMin=[]  NParamMax=[]  KbParamMin=[]  KbParamMax=[]  KtParamMin=[]  KtParamMax=[]  KbOutMin=[]  KbOutMax=[]  KtOutMin=[]  KtOutMax=[]  IntegratorOutMin=[]  IntegratorOutMax=[]  FilterOutMin=[]  FilterOutMax=[]  SumI1OutMin=[]  SumI1OutMax=[]  SumI2OutMin=[]  SumI2OutMax=[]  SumI3OutMin=[]  SumI3OutMax=[]  SumI4OutMin=[]  SumI4OutMax=[]  SumDOutMin=[]  SumDOutMax=[]  DifferentiatorOutMin=[]  DifferentiatorOutMax=[]  FilterDiffOutCoefMin=[]  FilterDiffOutCoefMax=[]  ReciprocalOutMin=[]  ReciprocalOutMax=[]  SumDenOutMin=[]  SumDenOutMax=[]  SumNumOutMin=[]  SumNumOutMax=[]  DivideOutMin=[]  DivideOutMax=[]  UdiffTsProdOutMin=[]  UdiffTsProdOutMax=[]  NTsProdOutMin=[]  NTsProdOutMax=[]  UintegralTsProdOutMin=[]  UintegralTsProdOutMax=[]  UngainTsProdOutMin=[]  UngainTsProdOutMax=[]  ClampingZeroOutDataTypeStr=Inherit: Inherit via back propagation  ClampingZeroOutMin=[]  ClampingZeroOutMax=[]  FilterDenConstantOutDataTypeStr=Inherit: Inherit via back propagation  FilterDenConstantOutMin=[]  FilterDenConstantOutMax=[]  PCopyOutDataTypeStr=Inherit: Inherit via back propagation  PCopyOutMin=[]  PCopyOutMax=[]  NCopyOutDataTypeStr=Inherit: Inherit via back propagation  NCopyOutMin=[]  NCopyOutMax=[]  IntegratorContinuousStateAttributes=''  IntegratorStateMustResolveToSignalObject=off  IntegratorRTWStateStorageClass=Auto  FilterContinuousStateAttributes=''  FilterStateMustResolveToSignalObject=off  FilterRTWStateStorageClass=Auto  ParallelPVariant=InternalParameters  IdealPVariant=Disabled  IVariant=InternalParameters  DVariant=Disabled  IntegratorVariant=Continuous  SatVariant=Disabled  AWVariant=Passthrough  PCopyVariant=Disabled  TRVariant=Disabled  FdbkBlocksVariant=Forward  IdealPFdbkVariant=Disabled  SatFdbkVariant=Disabled  DerivativeFilterVariant=Disabled  NVariant=Disabled  NCopyVariant=Disabled_SignalSpec  FilterICVariant=Disabled  IntegratorICVariant=InternalICs  ExternalResetVariant=Disabled  TRSumVariant=Passthrough  SumFdbkVariant=Disabled  SumVariant=Sum_PI  TsampFilterVariant=InternalTs  TsampNgainVariant=Passthrough  TsampIntegralVariant=Disabled_SignalSpec  ExternalSaturationOutDataTypeStr=Inherit: Same as second input  DerivativeSourceVariant=Disabled  PreIntVariant=InternalPreInt
  ParkClarke : MATLAB Function  TreatAsAtomicUnit=on
  Product : Product
  Selector : Selector  InputPortWidth=5  IndexOptions=Index vector (dialog)  Indices=[5]  OutputSizes=1
  Selector1 : Selector  InputPortWidth=5  IndexOptions=Index vector (dialog)  Indices=[4]  OutputSizes=1
  Selector2 : Selector  InputPortWidth=5  IndexOptions=Index vector (dialog)  Indices=[1:3]  OutputSizes=1
  Selector3 : Selector  InputPortWidth=5  IndexOptions=Index vector (dialog)  Indices=[4]  OutputSizes=1
  To File : ToFile  Commented=on  Filename=SimData\SteeringVabc.mat  SaveFormat=Timeseries
  Unit Delay : UnitDelay  InitialCondition=[0;0]  SampleTime=-1  HasFrameUpgradeWarning=on
  Vabc : Scope  Commented=on  NumInputPorts=3
  Wm_abc : Scope  Commented=on
  theta_m : Outport
  dWm : Outport  Port=2
  Wm : Outport  Port=3
  wires:
  Constant4/1 -> Add3/1  "i_d_ref"
  Back EMF/1(Fabc) -> BLDC abc model/2(f)
  Unit Delay/1 -> Demux1/1
  Add11/1 -> PID Controller6/1, [err_PI2]
  Add9/1 -> [err_PI1], PID Controller10/1
  Demux1/2 -> [I_q], Add4/2
  [Wm_abc] -> Add11/2
  [Theta_abc] -> Add9/2
  Selector2/1 -> ParkClarke/1(X_abc), I_abc/1, [I_abc]  "I_abc"
  Mux1/1 -> InvParkClarke/1(X_dq)
  [Theta_abc] -> ParkClarke/2(theta)
  [Theta_abc] -> InvParkClarke/2(theta)
  Selector/1 -> [Theta_abc], Divide/1  "Theta_abc"
  PID Controller3/1 -> Mux1/1
  ParkClarke/1(Y_dq) -> Unit Delay/1
  Tl/1 -> BLDC abc model/4(Tl)
  InvParkClarke/1(Y_abc) -> BLDC abc model/3(v), To File/1, Demux2/1  "Vabc"
  PID Controller4/1 -> Mux1/2
  BLDC abc model/1(dX) -> Selector3/1, Integrator2/1
  Selector1/1 -> Wm/1, [Wm_abc], Wm_abc/1  "Wm_abc"
  Add4/1 -> [err_PI3], PID Controller4/1
  Demux1/1 -> [I_d], Add3/2
  Add3/1 -> PID Controller3/1, [err_PI4]
  Integrator2/1 -> BLDC abc model/1(X), Back EMF/1(X), Selector/1, Selector2/1, Selector1/1
  [i_q_ref] -> Add4/1
  Product/1 -> Add9/1
  dd_ref/1 -> Product/1  "dd_ref"
  Constant2/1 -> Product/2
  Divide/1 -> theta_m/1
  Constant3/1 -> Divide/2
  [err_PI1] -> PI errors/1
  [err_PI2] -> PI errors/2
  [err_PI3] -> PI errors/3
  [err_PI4] -> PI errors/4
  Demux2/1 -> Vabc/1
  Demux2/2 -> Vabc/2
  Demux2/3 -> Vabc/3
  PID Controller6/1 -> [i_q_ref]  "i_q_ref"
  PID Controller10/1 -> Add11/1  "i_d_ref"
  Selector3/1 -> dWm/1  "Wm_abc"
  [I_d] -> Idq/1
  [I_q] -> Idq/2

== system LongLatDriveline/SteerActuator/BLDCWRack/RackSubsystem ==
  theta_m : Inport
  dWm : Inport  Port=2
  Wm : Inport  Port=3
  gearboxRate : Inport  Port=4
  Vx : Inport  Port=5
  Divide{,1..3} (4 alike) : Product  Inputs=*/
  Scope : Scope  NumInputPorts=3
  SteerMechanics : MATLAB Function  TreatAsAtomicUnit=on
  dd : Outport
  Tl : Outport  Port=2
  wires:
  theta_m/1 -> Divide/1  "delta"
  gearboxRate/1 -> Divide2/2, Divide1/2, Divide/2, Divide3/2  "Nm"
  dWm/1 -> Divide1/1
  Wm/1 -> Divide2/1
  Divide/1 -> dd/1, SteerMechanics/1(dd)
  Divide1/1 -> SteerMechanics/2(dWs)
  Divide2/1 -> SteerMechanics/3(Ws)
  SteerMechanics/1(Ts) -> Divide3/1  "Ts"
  Divide3/1 -> Scope/3, Tl/1  "Tl"
  SteerMechanics/2(t_f) -> Scope/1  "t_f"
  SteerMechanics/3(t_a) -> Scope/2  "t_a"
  Vx/1 -> SteerMechanics/4(Vx)  "Nm"

== system LongLatDriveline/Vehicle Lateral Model/DynamicModel/CoordConvertRotation ==
  note: dx and dy represents the longitudinal and lateral velocities, and psi is the yaw angle of the vehicle. in order to obtain the global coordinates (inertial reference frame) we need to convert the velocities from the G.C. reference of the vehicle to velocities in the inertial frame. afterwards integrate them.
  dx : Inport
  dy : Inport  Port=2
  Psi : Inport  Port=3
  Demux : Demux  Outputs=2
  Integrator10 : Integrator  InitialCondition=InitialX
  Integrator4 : Integrator  InitialCondition=InitialY
  MATLAB Function : MATLAB Function  TreatAsAtomicUnit=on
  Mux : Mux  Inputs=2
  X : Outport  VectorParamsAs1DForOutWhenUnconnected=off
  Y : Outport  Port=2  VectorParamsAs1DForOutWhenUnconnected=off
  wires:
  Integrator10/1 -> X/1  "X"
  Integrator4/1 -> Y/1  "Y"
  Psi/1 -> MATLAB Function/2(theta)
  dx/1 -> Mux/1
  dy/1 -> Mux/2
  Mux/1 -> MATLAB Function/1(A)
  MATLAB Function/1(B) -> Demux/1
  Demux/1 -> Integrator10/1
  Demux/2 -> Integrator4/1

== system LongLatDriveline/Vehicle Lateral Model/DynamicModel/LateralDynamics ==
  note: This variant does not simplify the small angle tan. i.e. tan(x) = x
  note: This variant does simplify the small angle tan. i.e. tan(x) = x
  note: This variant add disturbances to the dynamics. These can be modified inside.
  X : Inport
  Vx : Inport  Port=2
  dd : Inport  Port=3
  phi_ref : Inport  Port=4
  LateralDynamic : MATLAB Function  TreatAsAtomicUnit=on  VariantControl=Simplified Model
  LateralDynamic2 : MATLAB Function  TreatAsAtomicUnit=on  VariantControl=Not Simplified Model
  LateralDynamicWithNoise : Subsystem  VariantControl=Lateral dynamic with disturbances
      mask Display: image('$imagefile'); % Use "Edit Image" on toolstrip to change.
  dX : Outport

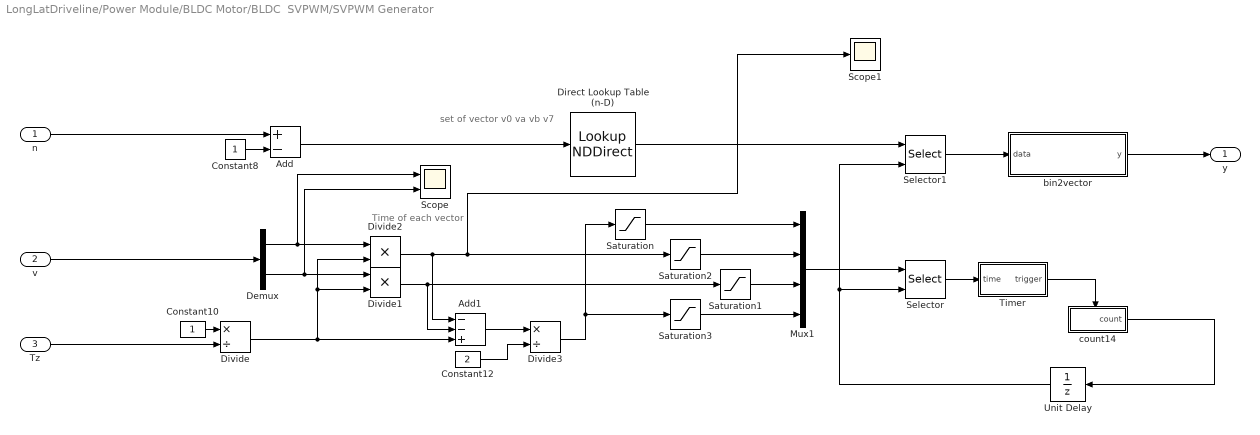
== system LongLatDriveline/Power Module/BLDC Motor/BLDC  SVPWM/SVPWM Generator ==
  note: set of vector v0 va vb v7
  note: Time of each vector
  n : Inport
  v : Inport  Port=2
  Tz : Inport  Port=3
  Add : Sum  Inputs=+-
  Add1 : Sum  Inputs=--+
  Constant10 : Constant
  Constant12 : Constant  Value=2
  Constant8 : Constant
  Demux : Demux  Outputs=2
  Direct Lookup Table (n-D) : LookupNDDirect  InputsSelectThisObjectFromTable=Vector  Table=[0 1 3 7;0 3 2 7;0 2 6 7;0 6 4 7; 0 4 5 7;0 5 1 7]'
  Divide : Product  Inputs=*/
  Divide1 : Product  Inputs=**
  Divide2 : Product  Inputs=**
  Divide3 : Product  Inputs=*/
  Mux1 : Mux
  Saturation{,1..3} (4 alike) : Saturate  UpperLimit=10000000  LowerLimit=0.00005
  Scope : Scope  NumInputPorts=2
  Scope1 : Scope
  Selector : Selector  InputPortWidth=4  IndexOptions=Index vector (port)  Indices=[1 3]  OutputSizes=1
  Selector1 : Selector  InputPortWidth=4  IndexOptions=Index vector (port)  Indices=[1 3]  OutputSizes=1
  Timer : Subsystem
  Unit Delay : UnitDelay  InitialCondition=1  SampleTime=-1  HasFrameUpgradeWarning=on
  bin2vector : MATLAB Function  TreatAsAtomicUnit=on
  count14 : Subsystem  TreatAsAtomicUnit=on
  y : Outport
  wires:
  Constant10/1 -> Divide/1
  Divide3/1 -> Saturation3/1, Saturation/1
  Divide1/1 -> Add1/2, Saturation1/1
  Constant8/1 -> Add/2
  v/1 -> Demux/1
  Divide2/1 -> Add1/1, Scope1/1, Saturation2/1
  Add/1 -> Direct Lookup Table (n-D)/1
  Divide/1 -> Divide1/2, Divide2/2, Add1/3
  count14/1(count) -> Unit Delay/1
  bin2vector/1(y) -> y/1
  Add1/1 -> Divide3/1
  Demux/2 -> Scope/2, Divide1/1
  Direct Lookup Table (n-D)/1 -> Selector1/1
  Demux/1 -> Scope/1, Divide2/1
  Constant12/1 -> Divide3/2
  Mux1/1 -> Selector/1
  n/1 -> Add/1
  Unit Delay/1 -> Selector1/2, Selector/2
  Selector/1 -> Timer/1(time)
  Timer/1(trigger) -> count14/Trigger
  Selector1/1 -> bin2vector/1(data)
  Tz/1 -> Divide/2
  Saturation/1 -> Mux1/1
  Saturation3/1 -> Mux1/4
  Saturation1/1 -> Mux1/3
  Saturation2/1 -> Mux1/2
